simulink model "PM_fnc18_Xload_duration_1Dlookup_TestHarness"  (R2022a)
settings: Solver=VariableStepAuto  StartTime=0.0  StopTime=inf  RelTol=1e-3
settings Model: Creator=306427  LastModifiedBy=306427

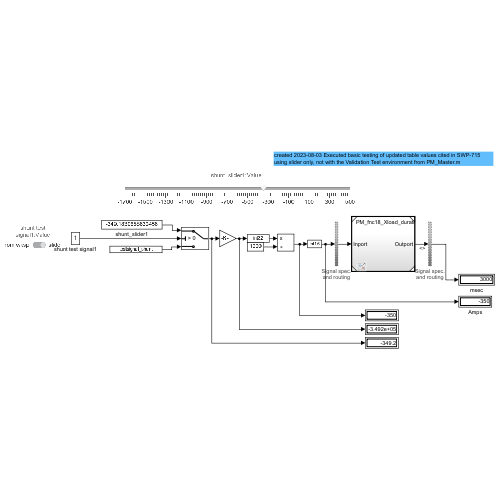
[thumbnail: Simulink's stored preview of the top-level diagram]
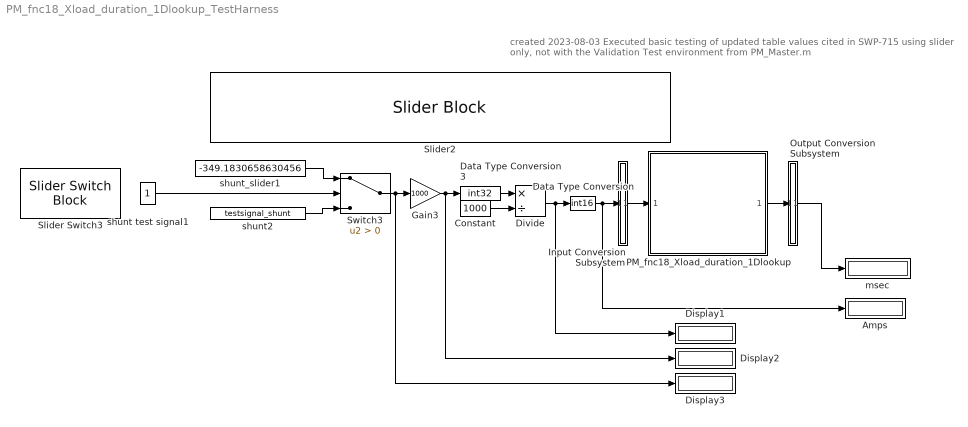
== system PM_fnc18_Xload_duration_1Dlookup_TestHarness ==
  note: created 2023-08-03 Executed basic testing of updated table values cited in SWP-715 using slider only, not with the Validation Test environment from PM_Master.m
  Amps : Display
  Constant : Constant  Value=1000
  Data Type Conversion : DataTypeConversion  OutDataTypeStr=int16  SaturateOnIntegerOverflow=off  RndMeth=Floor
  Data Type Conversion3 : DataTypeConversion  OutDataTypeStr=int32  SaturateOnIntegerOverflow=off  RndMeth=Floor
  Display1 : Display
  Display2 : Display
  Display3 : Display
  Divide : Product  Inputs=*/  OutDataTypeStr=int32  SaturateOnIntegerOverflow=on
  Gain3 : Gain  Gain=1000
  Input Conversion Subsystem : Subsystem  Tag=__SLT_ICS__  Description=|
      | Signal spec.
      | and routing
      settings: AttributesFormatString=%<Description>
  Output Conversion Subsystem : Subsystem  Tag=__SLT_OCS__  Description=|
      | Signal spec.
      | and routing
      settings: AttributesFormatString=%<Description>
  PM_fnc18_Xload_duration_1Dlookup : ModelReference  ModelNameDialog=PM_fnc18_Xload_duration_1Dlookup  SimulationMode=Normal  ModelReferenceVersion=1.4
  Slider Switch3 : SliderSwitchBlock
      settings: Values={{'from wksp', 'slider'}, [0 1]}
  Slider2 : SliderBlock  ScaleMin=-1700  ScaleMax=+500
  Switch3 : Switch  Criteria=u2 > Threshold  SaturateOnIntegerOverflow=off  InputSameDT=off
  msec : Display
  shunt test signal1 : Constant
  shunt2 : FromWorkspace  VariableName=testsignal_shunt  OutDataTypeStr=double
  shunt_slider1 : Constant  Value=-349.1830658630456  OutDataTypeStr=double
  wires:
  Output Conversion Subsystem/1(Outport_1) -> msec/1
  Data Type Conversion3/1 -> Divide/1
  Divide/1 -> Display1/1, Data Type Conversion/1
  Constant/1 -> Divide/2
  Data Type Conversion/1 -> Amps/1, Input Conversion Subsystem/1(Inport_1)
  shunt_slider1/1 -> Switch3/1
  Gain3/1 -> Display2/1, Data Type Conversion3/1
  shunt2/1 -> Switch3/3
  Switch3/1 -> Display3/1, Gain3/1
  shunt test signal1/1 -> Switch3/2
  PM_fnc18_Xload_duration_1Dlookup/1 -> Output Conversion Subsystem/1(Inport_1)
  Input Conversion Subsystem/1(Outport_1) -> PM_fnc18_Xload_duration_1Dlookup/1

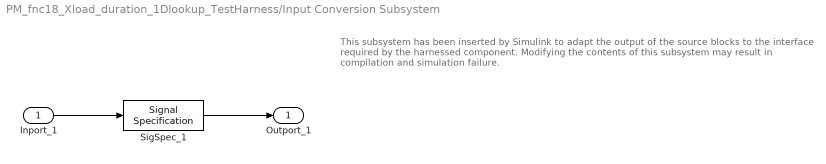
== system PM_fnc18_Xload_duration_1Dlookup_TestHarness/Input Conversion Subsystem ==
  note: This subsystem has been inserted by Simulink to adapt the output of the source blocks to the interface required by the harnessed component.
      |  Modifying the contents of this subsystem may result in compilation and simulation failure.
  Inport_1 : Inport
  SigSpec_1 : SignalSpecification  OutDataTypeStr=int16  Dimensions=[1]  SampleTime=[0, 0]
  Outport_1 : Outport
  wires:
  SigSpec_1/1 -> Outport_1/1
  Inport_1/1 -> SigSpec_1/1

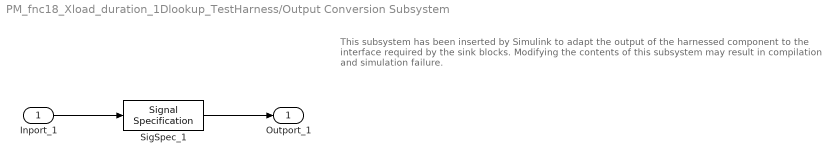
== system PM_fnc18_Xload_duration_1Dlookup_TestHarness/Output Conversion Subsystem ==
  note: This subsystem has been inserted by Simulink to adapt the output of the harnessed component to the interface required by the sink blocks.
      |  Modifying the contents of this subsystem may result in compilation and simulation failure.
  Inport_1 : Inport
  SigSpec_1 : SignalSpecification  OutDataTypeStr=uint32  Dimensions=[1]
  Outport_1 : Outport
  wires:
  Inport_1/1 -> SigSpec_1/1
  SigSpec_1/1 -> Outport_1/1
